simulink model "Plateforme_Stewart_fermeture_geometrique"  (R2019b)
settings: Solver=VariableStepAuto  StartTime=0.0  StopTime=10.0  RelTol=1e-3
PreLoadFcn:
  | addpath('Simscape')
model workspace (MATLAB code in the model file):
  | % Simscape(TM) Multibody(TM) version: 7.0
  | 
  | % This is a model data file derived from a Simscape Multibody Import XML file using the smimport function.
  | % The data in this file sets the block parameter values in an imported Simscape Multibody model.
  | % For more information on this file, see the smimport function help page in the Simscape Multibody documentation.
  | % You can modify numerical values, but avoid any other changes to this file.
  | % Do not add code to this file. Do not edit the physical units shown in comments.
  | 
  | %%%VariableName:smiData
  | 
  | 
  | %============= RigidTransform =============%
  | 
  | %Initialize the RigidTransform structure array by filling in null values.
  | smiData.RigidTransform(118).translation = [0.0 0.0 0.0];
  | smiData.RigidTransform(118).angle = 0.0;
  | smiData.RigidTransform(118).axis = [0.0 0.0 0.0];
  | smiData.RigidTransform(118).ID = '';
  | 
  | %Translation Method - Cartesian
  | %Rotation Method - Arbitrary Axis
  | smiData.RigidTransform(1).translation = [-109.40044094211088 0 0];  % mm
  | smiData.RigidTransform(1).angle = 0;  % rad
  | smiData.RigidTransform(1).axis = [0 0 0];
  | smiData.RigidTransform(1).ID = 'B[tige_verin-1:-:table_pltf-1]';
  | 
  | %Translation Method - Cartesian
  | %Rotation Method - Arbitrary Axis
  | smiData.RigidTransform(2).translation = [-577.50595932455826 -145.286666388404 9.0000000000001101];  % mm
  | smiData.RigidTransform(2).angle = 0;  % rad
  | smiData.RigidTransform(2).axis = [0 0 0];
  | smiData.RigidTransform(2).ID = 'F[tige_verin-1:-:table_pltf-1]';
  | 
  | %Translation Method - Cartesian
  | %Rotation Method - Arbitrary Axis
  | smiData.RigidTransform(3).translation = [-109.40044094211093 0 0];  % mm
  | smiData.RigidTransform(3).angle = 0;  % rad
  | smiData.RigidTransform(3).axis = [0 0 0];
  | smiData.RigidTransform(3).ID = 'B[tige_verin-2:-:table_pltf-1]';
  | 
  | %Translation Method - Cartesian
  | %Rotation Method - Arbitrary Axis
  | smiData.RigidTransform(4).translation = [-418.63100558659301 129.892825535908 9.0000000000000355];  % mm
  | smiData.RigidTransform(4).angle = 0;  % rad
  | smiData.RigidTransform(4).axis = [0 0 0];
  | smiData.RigidTransform(4).ID = 'F[tige_verin-2:-:table_pltf-1]';
  | 
  | %Translation Method - Cartesian
  | %Rotation Method - Arbitrary Axis
  | smiData.RigidTransform(5).translation = [-109.40044094211082 0 0];  % mm
  | smiData.RigidTransform(5).angle = 0;  % rad
  | smiData.RigidTransform(5).axis = [0 0 0];
  | smiData.RigidTransform(5).ID = 'B[tige_verin-4:-:table_pltf-1]';
  | 
  | %Translation Method - Cartesian
  | %Rotation Method - Arbitrary Axis
  | smiData.RigidTransform(6).translation = [-378.63100558659278 129.892825535908 9.0000000000002593];  % mm
  | smiData.RigidTransform(6).angle = 0;  % rad
  | smiData.RigidTransform(6).axis = [0 0 0];
  | smiData.RigidTransform(6).ID = 'F[tige_verin-4:-:table_pltf-1]';
  | 
  | %Translation Method - Cartesian
  | %Rotation Method - Arbitrary Axis
  | smiData.RigidTransform(7).translation = [-109.40044094211088 0 0];  % mm
  | smiData.RigidTransform(7).angle = 0;  % rad
  | smiData.RigidTransform(7).axis = [0 0 0];
  | smiData.RigidTransform(7).ID = 'B[tige_verin-5:-:table_pltf-1]';
  | 
  | %Translation Method - Cartesian
  | %Rotation Method - Arbitrary Axis
  | smiData.RigidTransform(8).translation = [-219.75605184862661 -145.28666638840158 9.0000000000000586];  % mm
  | smiData.RigidTransform(8).angle = 0;  % rad
  | smiData.RigidTransform(8).axis = [0 0 0];
  | smiData.RigidTransform(8).ID = 'F[tige_verin-5:-:table_pltf-1]';
  | 
  | %Translation Method - Cartesian
  | %Rotation Method - Arbitrary Axis
  | smiData.RigidTransform(9).translation = [-109.40044094211088 0 0];  % mm
  | smiData.RigidTransform(9).angle = 0;  % rad
  | smiData.RigidTransform(9).axis = [0 0 0];
  | smiData.RigidTransform(9).ID = 'B[tige_verin-6:-:table_pltf-1]';
  | 
  | %Translation Method - Cartesian
  | %Rotation Method - Arbitrary Axis
  | smiData.RigidTransform(10).translation = [-239.7560518486261 -179.92768253977937 9.0000000000000817];  % mm
  | smiData.RigidTransform(10).angle = 0;  % rad
  | smiData.RigidTransform(10).axis = [0 0 0];
  | smiData.RigidTransform(10).ID = 'F[tige_verin-6:-:table_pltf-1]';
  | 
  | %Translation Method - Cartesian
  | %Rotation Method - Arbitrary Axis
  | smiData.RigidTransform(11).translation = [-109.40044094211082 0 0];  % mm
  | smiData.RigidTransform(11).angle = 0;  % rad
  | smiData.RigidTransform(11).axis = [0 0 0];
  | smiData.RigidTransform(11).ID = 'B[tige_verin-7:-:table_pltf-1]';
  | 
  | %Translation Method - Cartesian
  | %Rotation Method - Arbitrary Axis
  | smiData.RigidTransform(12).translation = [-557.50595932455781 -179.92768253978147 9.0000000000000728];  % mm
  | smiData.RigidTransform(12).angle = 0;  % rad
  | smiData.RigidTransform(12).axis = [0 0 0];
  | smiData.RigidTransform(12).ID = 'F[tige_verin-7:-:table_pltf-1]';
  | 
  | %Translation Method - Cartesian
  | %Rotation Method - Arbitrary Axis
  | smiData.RigidTransform(13).translation = [0 0 0];  % mm
  | smiData.RigidTransform(13).angle = 0;  % rad
  | smiData.RigidTransform(13).axis = [0 0 0];
  | smiData.RigidTransform(13).ID = 'B[embase_pltf-1:-:]';
  | 
  | %Translation Method - Cartesian
  | %Rotation Method - Arbitrary Axis
  | smiData.RigidTransform(14).translation = [0 0 0];  % mm
  | smiData.RigidTransform(14).angle = 3.1415926535897931;  % rad
  | smiData.RigidTransform(14).axis = [2.4146537633967791e-16 -1 1.716137840753504e-16];
  | smiData.RigidTransform(14).ID = 'F[embase_pltf-1:-:]';
  | 
  | %Translation Method - Cartesian
  | %Rotation Method - Arbitrary Axis
  | smiData.RigidTransform(15).translation = [-21.777181335342689 270.78500270056696 -10.421088649404936];  % mm
  | smiData.RigidTransform(15).angle = 0;  % rad
  | smiData.RigidTransform(15).axis = [0 0 0];
  | smiData.RigidTransform(15).ID = 'B[embase_pltf-1:-:corps_verin-1]';
  | 
  | %Translation Method - Cartesian
  | %Rotation Method - Arbitrary Axis
  | smiData.RigidTransform(16).translation = [-402.58704714007331 -133.73646344618052 13.096795646989449];  % mm
  | smiData.RigidTransform(16).angle = 0;  % rad
  | smiData.RigidTransform(16).axis = [0 0 0];
  | smiData.RigidTransform(16).ID = 'F[embase_pltf-1:-:corps_verin-1]';
  | 
  | %Translation Method - Cartesian
  | %Rotation Method - Arbitrary Axis
  | smiData.RigidTransform(17).translation = [20.111591903521756 272.65573361842087 -6.7232809872821688];  % mm
  | smiData.RigidTransform(17).angle = 0;  % rad
  | smiData.RigidTransform(17).axis = [0 0 0];
  | smiData.RigidTransform(17).ID = 'B[embase_pltf-1:-:corps_verin-2]';
  | 
  | %Translation Method - Cartesian
  | %Rotation Method - Arbitrary Axis
  | smiData.RigidTransform(18).translation = [-402.58704714007342 -133.73646344618064 13.096795646989392];  % mm
  | smiData.RigidTransform(18).angle = 0;  % rad
  | smiData.RigidTransform(18).axis = [0 0 0];
  | smiData.RigidTransform(18).ID = 'F[embase_pltf-1:-:corps_verin-2]';
  | 
  | %Translation Method - Cartesian
  | %Rotation Method - Arbitrary Axis
  | smiData.RigidTransform(19).translation = [246.18258775279722 -118.91071731021286 -6.7232809872821191];  % mm
  | smiData.RigidTransform(19).angle = 0;  % rad
  | smiData.RigidTransform(19).axis = [0 0 0];
  | smiData.RigidTransform(19).ID = 'B[embase_pltf-1:-:corps_verin-3]';
  | 
  | %Translation Method - Cartesian
  | %Rotation Method - Arbitrary Axis
  | smiData.RigidTransform(20).translation = [-402.58704714007342 -133.73646344617663 13.096795646991893];  % mm
  | smiData.RigidTransform(20).angle = 0;  % rad
  | smiData.RigidTransform(20).axis = [0 0 0];
  | smiData.RigidTransform(20).ID = 'F[embase_pltf-1:-:corps_verin-3]';
  | 
  | %Translation Method - Cartesian
  | %Rotation Method - Arbitrary Axis
  | smiData.RigidTransform(21).translation = [226.07099584927582 -153.74501630820362 -6.7232809872821164];  % mm
  | smiData.RigidTransform(21).angle = 0;  % rad
  | smiData.RigidTransform(21).axis = [0 0 0];
  | smiData.RigidTransform(21).ID = 'B[embase_pltf-1:-:corps_verin-4]';
  | 
  | %Translation Method - Cartesian
  | %Rotation Method - Arbitrary Axis
  | smiData.RigidTransform(22).translation = [-402.58704714007337 -133.73646344617981 13.096795646989108];  % mm
  | smiData.RigidTransform(22).angle = 0;  % rad
  | smiData.RigidTransform(22).axis = [0 0 0];
  | smiData.RigidTransform(22).ID = 'F[embase_pltf-1:-:corps_verin-4]';
  | 
  | %Translation Method - Cartesian
  | %Rotation Method - Arbitrary Axis
  | smiData.RigidTransform(23).translation = [-226.07099584927371 -153.74501630820677 -6.7232809872821617];  % mm
  | smiData.RigidTransform(23).angle = 0;  % rad
  | smiData.RigidTransform(23).axis = [0 0 0];
  | smiData.RigidTransform(23).ID = 'B[embase_pltf-1:-:corps_verin-5]';
  | 
  | %Translation Method - Cartesian
  | %Rotation Method - Arbitrary Axis
  | smiData.RigidTransform(24).translation = [-402.58704714007354 -133.73646344618081 13.096795646989619];  % mm
  | smiData.RigidTransform(24).angle = 0;  % rad
  | smiData.RigidTransform(24).axis = [0 0 0];
  | smiData.RigidTransform(24).ID = 'F[embase_pltf-1:-:corps_verin-5]';
  | 
  | %Translation Method - Cartesian
  | %Rotation Method - Arbitrary Axis
  | smiData.RigidTransform(25).translation = [-246.18258775279565 -118.91071731021631 -6.7232809872821564];  % mm
  | smiData.RigidTransform(25).angle = 0;  % rad
  | smiData.RigidTransform(25).axis = [0 0 0];
  | smiData.RigidTransform(25).ID = 'B[embase_pltf-1:-:corps_verin-6]';
  | 
  | %Translation Method - Cartesian
  | %Rotation Method - Arbitrary Axis
  | smiData.RigidTransform(26).translation = [-402.58704714007354 -133.73646344618049 13.096795646989506];  % mm
  | smiData.RigidTransform(26).angle = 0;  % rad
  | smiData.RigidTransform(26).axis = [0 0 0];
  | smiData.RigidTransform(26).ID = 'F[embase_pltf-1:-:corps_verin-6]';
  | 
  | %Translation Method - Cartesian
  | %Rotation Method - Arbitrary Axis
  | smiData.RigidTransform(27).translation = [-258.58704714007337 -133.73646344618055 13.096795646989408];  % mm
  | smiData.RigidTransform(27).angle = 2.0943951023931953;  % rad
  | smiData.RigidTransform(27).axis = [-0.57735026918962584 -0.57735026918962584 0.57735026918962584];
  | smiData.RigidTransform(27).ID = 'B[corps_verin-1:-:tige_verin-1]';
  | 
  | %Translation Method - Cartesian
  | %Rotation Method - Arbitrary Axis
  | smiData.RigidTransform(28).translation = [-392.59341329234132 -3.1263880373444408e-13 1.1368683772161603e-13];  % mm
  | smiData.RigidTransform(28).angle = 2.0943951023931962;  % rad
  | smiData.RigidTransform(28).axis = [-0.57735026918962562 -0.57735026918962595 0.57735026918962573];
  | smiData.RigidTransform(28).ID = 'F[corps_verin-1:-:tige_verin-1]';
  | 
  | %Translation Method - Cartesian
  | %Rotation Method - Arbitrary Axis
  | smiData.RigidTransform(29).translation = [-258.58704714007342 -133.73646344618055 13.096795646989484];  % mm
  | smiData.RigidTransform(29).angle = 2.0943951023931953;  % rad
  | smiData.RigidTransform(29).axis = [-0.57735026918962584 -0.57735026918962584 0.57735026918962584];
  | smiData.RigidTransform(29).ID = 'B[corps_verin-2:-:tige_verin-2]';
  | 
  | %Translation Method - Cartesian
  | %Rotation Method - Arbitrary Axis
  | smiData.RigidTransform(30).translation = [-392.59341329234149 4.2632564145606011e-13 2.2737367544323206e-13];  % mm
  | smiData.RigidTransform(30).angle = 2.0943951023931944;  % rad
  | smiData.RigidTransform(30).axis = [-0.57735026918962595 -0.57735026918962529 0.57735026918962595];
  | smiData.RigidTransform(30).ID = 'F[corps_verin-2:-:tige_verin-2]';
  | 
  | %Translation Method - Cartesian
  | %Rotation Method - Arbitrary Axis
  | smiData.RigidTransform(31).translation = [-258.58704714007342 -133.73646344618058 13.096795646989456];  % mm
  | smiData.RigidTransform(31).angle = 2.0943951023931953;  % rad
  | smiData.RigidTransform(31).axis = [-0.57735026918962584 -0.57735026918962584 0.57735026918962584];
  | smiData.RigidTransform(31).ID = 'B[corps_verin-3:-:tige_verin-4]';
  | 
  | %Translation Method - Cartesian
  | %Rotation Method - Arbitrary Axis
  | smiData.RigidTransform(32).translation = [-392.59341329234132 -4.2916781239910051e-12 1.0231815394945443e-12];  % mm
  | smiData.RigidTransform(32).angle = 2.0943951023931953;  % rad
  | smiData.RigidTransform(32).axis = [-0.57735026918962629 -0.57735026918962584 0.57735026918962529];
  | smiData.RigidTransform(32).ID = 'F[corps_verin-3:-:tige_verin-4]';
  | 
  | %Translation Method - Cartesian
  | %Rotation Method - Arbitrary Axis
  | smiData.RigidTransform(33).translation = [-258.58704714007342 -133.73646344618061 13.096795646989429];  % mm
  | smiData.RigidTransform(33).angle = 2.0943951023931953;  % rad
  | smiData.RigidTransform(33).axis = [-0.57735026918962584 -0.57735026918962584 0.57735026918962584];
  | smiData.RigidTransform(33).ID = 'B[corps_verin-4:-:tige_verin-5]';
  | 
  | %Translation Method - Cartesian
  | %Rotation Method - Arbitrary Axis
  | smiData.RigidTransform(34).translation = [-392.59341329234155 8.6686213762732223e-13 6.8212102632969618e-13];  % mm
  | smiData.RigidTransform(34).angle = 2.0943951023931948;  % rad
  | smiData.RigidTransform(34).axis = [-0.57735026918962529 -0.57735026918962551 0.57735026918962662];
  | smiData.RigidTransform(34).ID = 'F[corps_verin-4:-:tige_verin-5]';
  | 
  | %Translation Method - Cartesian
  | %Rotation Method - Arbitrary Axis
  | smiData.RigidTransform(35).translation = [-258.58704714007331 -133.73646344618061 13.096795646989477];  % mm
  | smiData.RigidTransform(35).angle = 2.0943951023931953;  % rad
  | smiData.RigidTransform(35).axis = [-0.57735026918962584 -0.57735026918962584 0.57735026918962584];
  | smiData.RigidTransform(35).ID = 'B[corps_verin-5:-:tige_verin-6]';
  | 
  | %Translation Method - Cartesian
  | %Rotation Method - Arbitrary Axis
  | smiData.RigidTransform(36).translation = [-392.59341329234189 1.4210854715202004e-13 2.2737367544323206e-13];  % mm
  | smiData.RigidTransform(36).angle = 2.0943951023931953;  % rad
  | smiData.RigidTransform(36).axis = [-0.57735026918962618 -0.57735026918962562 0.5773502691896254];
  | smiData.RigidTransform(36).ID = 'F[corps_verin-5:-:tige_verin-6]';
  | 
  | %Translation Method - Cartesian
  | %Rotation Method - Arbitrary Axis
  | smiData.RigidTransform(37).translation = [-258.58704714007342 -133.73646344618055 13.096795646989401];  % mm
  | smiData.RigidTransform(37).angle = 2.0943951023931953;  % rad
  | smiData.RigidTransform(37).axis = [-0.57735026918962584 -0.57735026918962584 0.57735026918962584];
  | smiData.RigidTransform(37).ID = 'B[corps_verin-6:-:tige_verin-7]';
  | 
  | %Translation Method - Cartesian
  | %Rotation Method - Arbitrary Axis
  | smiData.RigidTransform(38).translation = [-392.59341329234144 1.9895196601282805e-13 -2.2737367544323206e-13];  % mm
  | smiData.RigidTransform(38).angle = 2.0943951023931953;  % rad
  | smiData.RigidTransform(38).axis = [-0.57735026918962595 -0.57735026918962562 0.57735026918962562];
  | smiData.RigidTransform(38).ID = 'F[corps_verin-6:-:tige_verin-7]';
  | 
  | %Translation Method - Cartesian
  | %Rotation Method - Arbitrary Axis
  | smiData.RigidTransform(39).translation = [-385.58704714007331 -133.73646344618061 13.096795646989415];  % mm
  | smiData.RigidTransform(39).angle = 0;  % rad
  | smiData.RigidTransform(39).axis = [0 0 0];
  | smiData.RigidTransform(39).ID = 'AssemblyGround[corps_verin-1:tube_inf-1]';
  | 
  | %Translation Method - Cartesian
  | %Rotation Method - Arbitrary Axis
  | smiData.RigidTransform(40).translation = [-385.58704714007342 -133.73646344618055 13.096795646989401];  % mm
  | smiData.RigidTransform(40).angle = 0;  % rad
  | smiData.RigidTransform(40).axis = [0 0 0];
  | smiData.RigidTransform(40).ID = 'AssemblyGround[corps_verin-1:embout_inf-1]';
  | 
  | %Translation Method - Cartesian
  | %Rotation Method - Arbitrary Axis
  | smiData.RigidTransform(41).translation = [-402.58704714007337 -133.73646344618055 13.096795646989394];  % mm
  | smiData.RigidTransform(41).angle = 0;  % rad
  | smiData.RigidTransform(41).axis = [0 0 0];
  | smiData.RigidTransform(41).ID = 'AssemblyGround[corps_verin-1:sphere-1]';
  | 
  | %Translation Method - Cartesian
  | %Rotation Method - Arbitrary Axis
  | smiData.RigidTransform(42).translation = [-271.58704714007337 -133.73646344618061 13.096795646989401];  % mm
  | smiData.RigidTransform(42).angle = 0;  % rad
  | smiData.RigidTransform(42).axis = [0 0 0];
  | smiData.RigidTransform(42).ID = 'AssemblyGround[corps_verin-1:boitier-1]';
  | 
  | %Translation Method - Cartesian
  | %Rotation Method - Arbitrary Axis
  | smiData.RigidTransform(43).translation = [-258.58704714007337 -133.73646344618055 13.096795646989408];  % mm
  | smiData.RigidTransform(43).angle = 0;  % rad
  | smiData.RigidTransform(43).axis = [0 0 0];
  | smiData.RigidTransform(43).ID = 'AssemblyGround[corps_verin-1:tube_sup-1]';
  | 
  | %Translation Method - Cartesian
  | %Rotation Method - Arbitrary Axis
  | smiData.RigidTransform(44).translation = [-271.58704714007337 -117.73646344618061 6.8467956469894027];  % mm
  | smiData.RigidTransform(44).angle = 1.5707963267948966;  % rad
  | smiData.RigidTransform(44).axis = [-1 -1.3877787807814457e-16 -1.3877787807814467e-16];
  | smiData.RigidTransform(44).ID = 'AssemblyGround[corps_verin-1:couvercle-1]';
  | 
  | %Translation Method - Cartesian
  | %Rotation Method - Arbitrary Axis
  | smiData.RigidTransform(45).translation = [-47.394074789842975 -133.73646344618061 13.096795646989456];  % mm
  | smiData.RigidTransform(45).angle = 3.1415926535897931;  % rad
  | smiData.RigidTransform(45).axis = [-2.851611096621234e-17 0.22941107115039033 0.97332962578647042];
  | smiData.RigidTransform(45).ID = 'AssemblyGround[corps_verin-1:palier-1]';
  | 
  | %Translation Method - Cartesian
  | %Rotation Method - Arbitrary Axis
  | smiData.RigidTransform(46).translation = [-121.40044094211083 0 0];  % mm
  | smiData.RigidTransform(46).angle = 3.1415926535897931;  % rad
  | smiData.RigidTransform(46).axis = [6.3638526192303913e-17 0.47606521271394214 0.87940998018195637];
  | smiData.RigidTransform(46).ID = 'AssemblyGround[tige_verin-7:embout_sup-1]';
  | 
  | %Translation Method - Cartesian
  | %Rotation Method - Arbitrary Axis
  | smiData.RigidTransform(47).translation = [-281.40044094211089 0 0];  % mm
  | smiData.RigidTransform(47).angle = 0.80510609664977162;  % rad
  | smiData.RigidTransform(47).axis = [-1 0 0];
  | smiData.RigidTransform(47).ID = 'AssemblyGround[tige_verin-7:tige-1]';
  | 
  | %Translation Method - Cartesian
  | %Rotation Method - Arbitrary Axis
  | smiData.RigidTransform(48).translation = [-286.40044094211095 0 0];  % mm
  | smiData.RigidTransform(48).angle = 0;  % rad
  | smiData.RigidTransform(48).axis = [0 0 0];
  | smiData.RigidTransform(48).ID = 'AssemblyGround[tige_verin-7:ecrou-1]';
  | 
  | %Translation Method - Cartesian
  | %Rotation Method - Arbitrary Axis
  | smiData.RigidTransform(49).translation = [-109.40044094211082 0 0];  % mm
  | smiData.RigidTransform(49).angle = 0;  % rad
  | smiData.RigidTransform(49).axis = [0 0 0];
  | smiData.RigidTransform(49).ID = 'AssemblyGround[tige_verin-7:sphere-1]';
  | 
  | %Translation Method - Cartesian
  | %Rotation Method - Arbitrary Axis
  | smiData.RigidTransform(50).translation = [-238.63105184862621 -177.9791253812642 5.1028856829702374];  % mm
  | smiData.RigidTransform(50).angle = 1.8452184908695632;  % rad
  | smiData.RigidTransform(50).axis = [0.12851178747769235 -0.94870612275177946 -0.28886227364017958];
  | smiData.RigidTransform(50).ID = 'AssemblyGround[table_pltf-1:ext_sph-6]';
  | 
  | %Translation Method - Cartesian
  | %Rotation Method - Arbitrary Axis
  | smiData.RigidTransform(51).translation = [-558.63095932455781 -177.97912538126641 5.1028856829702374];  % mm
  | smiData.RigidTransform(51).angle = 1.3181160716528153;  % rad
  | smiData.RigidTransform(51).axis = [8.5997505698985228e-17 -0.89442719099991586 -0.44721359549995787];
  | smiData.RigidTransform(51).ID = 'AssemblyGround[table_pltf-1:ext_sph-4]';
  | 
  | %Translation Method - Cartesian
  | %Rotation Method - Arbitrary Axis
  | smiData.RigidTransform(52).translation = [-416.38100558659278 129.89282553590814 5.1028856829702374];  % mm
  | smiData.RigidTransform(52).angle = 1.1138509682631477;  % rad
  | smiData.RigidTransform(52).axis = [-0.32436275744359122 0.92721000971271517 0.18727092532514639];
  | smiData.RigidTransform(52).ID = 'AssemblyGround[table_pltf-1:ext_sph-1]';
  | 
  | %Translation Method - Cartesian
  | %Rotation Method - Arbitrary Axis
  | smiData.RigidTransform(53).translation = [-220.88105184862647 -147.23522354691647 5.1028856829702924];  % mm
  | smiData.RigidTransform(53).angle = 1.4414924728059237;  % rad
  | smiData.RigidTransform(53).axis = [-0.37279524950071685 -0.91787977789370334 0.13608973246907444];
  | smiData.RigidTransform(53).ID = 'AssemblyGround[table_pltf-1:ext_sph-5]';
  | 
  | %Translation Method - Cartesian
  | %Rotation Method - Arbitrary Axis
  | smiData.RigidTransform(54).translation = [-380.88100558659272 129.89282553590814 5.1028856829703484];  % mm
  | smiData.RigidTransform(54).angle = 1.3047235338847067;  % rad
  | smiData.RigidTransform(54).axis = [-0.56711997758819543 -0.75575563159914327 -0.32742687172335888];
  | smiData.RigidTransform(54).ID = 'AssemblyGround[table_pltf-1:ext_sph-2]';
  | 
  | %Translation Method - Cartesian
  | %Rotation Method - Arbitrary Axis
  | smiData.RigidTransform(55).translation = [-576.38095932455803 -147.23522354691895 5.1028856829701823];  % mm
  | smiData.RigidTransform(55).angle = 1.5789537349491201;  % rad
  | smiData.RigidTransform(55).axis = [-0.5060320994735239 0.86248629273953803 0.006993506904675686];
  | smiData.RigidTransform(55).ID = 'AssemblyGround[table_pltf-1:ext_sph-3]';
  | 
  | %Translation Method - Cartesian
  | %Rotation Method - Arbitrary Axis
  | smiData.RigidTransform(56).translation = [-398.63100558659278 -65.107174464091898 -12.547005383792332];  % mm
  | smiData.RigidTransform(56).angle = 0;  % rad
  | smiData.RigidTransform(56).axis = [0 0 0];
  | smiData.RigidTransform(56).ID = 'AssemblyGround[table_pltf-1:table3-1]';
  | 
  | %Translation Method - Cartesian
  | %Rotation Method - Arbitrary Axis
  | smiData.RigidTransform(57).translation = [-385.58704714007331 -133.73646344618061 13.096795646989456];  % mm
  | smiData.RigidTransform(57).angle = 0;  % rad
  | smiData.RigidTransform(57).axis = [0 0 0];
  | smiData.RigidTransform(57).ID = 'AssemblyGround[corps_verin-3:tube_inf-1]';
  | 
  | %Translation Method - Cartesian
  | %Rotation Method - Arbitrary Axis
  | smiData.RigidTransform(58).translation = [-385.58704714007342 -133.73646344618061 13.096795646989456];  % mm
  | smiData.RigidTransform(58).angle = 0;  % rad
  | smiData.RigidTransform(58).axis = [0 0 0];
  | smiData.RigidTransform(58).ID = 'AssemblyGround[corps_verin-3:embout_inf-1]';
  | 
  | %Translation Method - Cartesian
  | %Rotation Method - Arbitrary Axis
  | smiData.RigidTransform(59).translation = [-402.58704714007337 -133.73646344618061 13.096795646989456];  % mm
  | smiData.RigidTransform(59).angle = 0;  % rad
  | smiData.RigidTransform(59).axis = [0 0 0];
  | smiData.RigidTransform(59).ID = 'AssemblyGround[corps_verin-3:sphere-1]';
  | 
  | %Translation Method - Cartesian
  | %Rotation Method - Arbitrary Axis
  | smiData.RigidTransform(60).translation = [-271.58704714007337 -133.73646344618058 13.096795646989484];  % mm
  | smiData.RigidTransform(60).angle = 0;  % rad
  | smiData.RigidTransform(60).axis = [0 0 0];
  | smiData.RigidTransform(60).ID = 'AssemblyGround[corps_verin-3:boitier-1]';
  | 
  | %Translation Method - Cartesian
  | %Rotation Method - Arbitrary Axis
  | smiData.RigidTransform(61).translation = [-258.58704714007342 -133.73646344618058 13.096795646989456];  % mm
  | smiData.RigidTransform(61).angle = 0;  % rad
  | smiData.RigidTransform(61).axis = [0 0 0];
  | smiData.RigidTransform(61).ID = 'AssemblyGround[corps_verin-3:tube_sup-1]';
  | 
  | %Translation Method - Cartesian
  | %Rotation Method - Arbitrary Axis
  | smiData.RigidTransform(62).translation = [-271.58704714007331 -117.73646344618059 6.8467956469894506];  % mm
  | smiData.RigidTransform(62).angle = 1.5707963267948966;  % rad
  | smiData.RigidTransform(62).axis = [-1 -9.7144514654701185e-17 -1.2490009027033011e-16];
  | smiData.RigidTransform(62).ID = 'AssemblyGround[corps_verin-3:couvercle-1]';
  | 
  | %Translation Method - Cartesian
  | %Rotation Method - Arbitrary Axis
  | smiData.RigidTransform(63).translation = [-47.394074789842975 -133.73646344618066 13.096795646989484];  % mm
  | smiData.RigidTransform(63).angle = 3.1415926535897931;  % rad
  | smiData.RigidTransform(63).axis = [3.1848379601679358e-17 0.22941107115039044 0.97332962578647042];
  | smiData.RigidTransform(63).ID = 'AssemblyGround[corps_verin-3:palier-1]';
  | 
  | %Translation Method - Cartesian
  | %Rotation Method - Arbitrary Axis
  | smiData.RigidTransform(64).translation = [-385.58704714007337 -133.73646344618064 13.096795646989429];  % mm
  | smiData.RigidTransform(64).angle = 0;  % rad
  | smiData.RigidTransform(64).axis = [0 0 0];
  | smiData.RigidTransform(64).ID = 'AssemblyGround[corps_verin-4:tube_inf-1]';
  | 
  | %Translation Method - Cartesian
  | %Rotation Method - Arbitrary Axis
  | smiData.RigidTransform(65).translation = [-385.58704714007348 -133.73646344618066 13.096795646989456];  % mm
  | smiData.RigidTransform(65).angle = 0;  % rad
  | smiData.RigidTransform(65).axis = [0 0 0];
  | smiData.RigidTransform(65).ID = 'AssemblyGround[corps_verin-4:embout_inf-1]';
  | 
  | %Translation Method - Cartesian
  | %Rotation Method - Arbitrary Axis
  | smiData.RigidTransform(66).translation = [-402.58704714007342 -133.73646344618061 13.096795646989456];  % mm
  | smiData.RigidTransform(66).angle = 0;  % rad
  | smiData.RigidTransform(66).axis = [0 0 0];
  | smiData.RigidTransform(66).ID = 'AssemblyGround[corps_verin-4:sphere-1]';
  | 
  | %Translation Method - Cartesian
  | %Rotation Method - Arbitrary Axis
  | smiData.RigidTransform(67).translation = [-271.58704714007337 -133.73646344618066 13.096795646989429];  % mm
  | smiData.RigidTransform(67).angle = 0;  % rad
  | smiData.RigidTransform(67).axis = [0 0 0];
  | smiData.RigidTransform(67).ID = 'AssemblyGround[corps_verin-4:boitier-1]';
  | 
  | %Translation Method - Cartesian
  | %Rotation Method - Arbitrary Axis
  | smiData.RigidTransform(68).translation = [-258.58704714007342 -133.73646344618061 13.096795646989429];  % mm
  | smiData.RigidTransform(68).angle = 0;  % rad
  | smiData.RigidTransform(68).axis = [0 0 0];
  | smiData.RigidTransform(68).ID = 'AssemblyGround[corps_verin-4:tube_sup-1]';
  | 
  | %Translation Method - Cartesian
  | %Rotation Method - Arbitrary Axis
  | smiData.RigidTransform(69).translation = [-271.58704714007337 -117.73646344618064 6.8467956469894231];  % mm
  | smiData.RigidTransform(69).angle = 1.5707963267948966;  % rad
  | smiData.RigidTransform(69).axis = [-1 -1.1796119636642288e-16 -2.4980018054066022e-16];
  | smiData.RigidTransform(69).ID = 'AssemblyGround[corps_verin-4:couvercle-1]';
  | 
  | %Translation Method - Cartesian
  | %Rotation Method - Arbitrary Axis
  | smiData.RigidTransform(70).translation = [-47.394074789843032 -133.73646344618066 13.096795646989429];  % mm
  | smiData.RigidTransform(70).angle = 3.1415926535897931;  % rad
  | smiData.RigidTransform(70).axis = [2.8516110966212334e-17 0.22941107115039044 0.97332962578647042];
  | smiData.RigidTransform(70).ID = 'AssemblyGround[corps_verin-4:palier-1]';
  | 
  | %Translation Method - Cartesian
  | %Rotation Method - Arbitrary Axis
  | smiData.RigidTransform(71).translation = [-121.40044094211089 0 0];  % mm
  | smiData.RigidTransform(71).angle = 3.1415926535897931;  % rad
  | smiData.RigidTransform(71).axis = [0 0.4760652127139422 0.8794099801819566];
  | smiData.RigidTransform(71).ID = 'AssemblyGround[tige_verin-5:embout_sup-1]';
  | 
  | %Translation Method - Cartesian
  | %Rotation Method - Arbitrary Axis
  | smiData.RigidTransform(72).translation = [-281.40044094211089 0 0];  % mm
  | smiData.RigidTransform(72).angle = 0.80510609664977162;  % rad
  | smiData.RigidTransform(72).axis = [-1 -2.5106205397484075e-16 7.700212191956017e-17];
  | smiData.RigidTransform(72).ID = 'AssemblyGround[tige_verin-5:tige-1]';
  | 
  | %Translation Method - Cartesian
  | %Rotation Method - Arbitrary Axis
  | smiData.RigidTransform(73).translation = [-286.40044094211095 0 0];  % mm
  | smiData.RigidTransform(73).angle = 0;  % rad
  | smiData.RigidTransform(73).axis = [0 0 0];
  | smiData.RigidTransform(73).ID = 'AssemblyGround[tige_verin-5:ecrou-1]';
  | 
  | %Translation Method - Cartesian
  | %Rotation Method - Arbitrary Axis
  | smiData.RigidTransform(74).translation = [-109.40044094211088 0 0];  % mm
  | smiData.RigidTransform(74).angle = 0;  % rad
  | smiData.RigidTransform(74).axis = [0 0 0];
  | smiData.RigidTransform(74).ID = 'AssemblyGround[tige_verin-5:sphere-1]';
  | 
  | %Translation Method - Cartesian
  | %Rotation Method - Arbitrary Axis
  | smiData.RigidTransform(75).translation = [0 0 0];  % mm
  | smiData.RigidTransform(75).angle = 0;  % rad
  | smiData.RigidTransform(75).axis = [0 0 0];
  | smiData.RigidTransform(75).ID = 'AssemblyGround[embase_pltf-1:embase-1]';
  | 
  | %Translation Method - Cartesian
  | %Rotation Method - Arbitrary Axis
  | smiData.RigidTransform(76).translation = [-20.111591903521784 272.65573361842087 -6.7232809872821715];  % mm
  | smiData.RigidTransform(76).angle = 1.1886358755650654;  % rad
  | smiData.RigidTransform(76).axis = [-2.3930801898784881e-16 -0.89231044576403895 0.45142227280051467];
  | smiData.RigidTransform(76).ID = 'AssemblyGround[embase_pltf-1:ext_sph-1]';
  | 
  | %Translation Method - Cartesian
  | %Rotation Method - Arbitrary Axis
  | smiData.RigidTransform(77).translation = [20.111591903521756 272.65573361842087 -6.7232809872821688];  % mm
  | smiData.RigidTransform(77).angle = 1.1886358755650657;  % rad
  | smiData.RigidTransform(77).axis = [2.9913502373481095e-17 0.89231044576403895 -0.45142227280051433];
  | smiData.RigidTransform(77).ID = 'AssemblyGround[embase_pltf-1:ext_sph-2]';
  | 
  | %Translation Method - Cartesian
  | %Rotation Method - Arbitrary Axis
  | smiData.RigidTransform(78).translation = [246.18258775279722 -118.91071731021286 -6.7232809872821191];  % mm
  | smiData.RigidTransform(78).angle = 1.3935923944935191;  % rad
  | smiData.RigidTransform(78).axis = [5.6394261391252521e-17 -0.84111161395084555 -0.54086158384285687];
  | smiData.RigidTransform(78).ID = 'AssemblyGround[embase_pltf-1:ext_sph-3]';
  | 
  | %Translation Method - Cartesian
  | %Rotation Method - Arbitrary Axis
  | smiData.RigidTransform(79).translation = [226.07099584927582 -153.74501630820362 -6.7232809872821164];  % mm
  | smiData.RigidTransform(79).angle = 0.98938499076868036;  % rad
  | smiData.RigidTransform(79).axis = [-2.9061226051580059e-17 -0.99072835303675166 0.13585775829552582];
  | smiData.RigidTransform(79).ID = 'AssemblyGround[embase_pltf-1:ext_sph-4]';
  | 
  | %Translation Method - Cartesian
  | %Rotation Method - Arbitrary Axis
  | smiData.RigidTransform(80).translation = [-246.18258775279565 -118.91071731021631 -6.7232809872821564];  % mm
  | smiData.RigidTransform(80).angle = 1.3937057673028201;  % rad
  | smiData.RigidTransform(80).axis = [-0.011638836419521733 0.83574692275854157 0.54899145584100639];
  | smiData.RigidTransform(80).ID = 'AssemblyGround[embase_pltf-1:ext_sph-6]';
  | 
  | %Translation Method - Cartesian
  | %Rotation Method - Arbitrary Axis
  | smiData.RigidTransform(81).translation = [-226.07099584927371 -153.74501630820677 -6.7232809872821617];  % mm
  | smiData.RigidTransform(81).angle = 0.98938499076867825;  % rad
  | smiData.RigidTransform(81).axis = [2.9061226051580096e-17 0.99072835303675288 -0.13585775829551691];
  | smiData.RigidTransform(81).ID = 'AssemblyGround[embase_pltf-1:ext_sph-5]';
  | 
  | %Translation Method - Cartesian
  | %Rotation Method - Arbitrary Axis
  | smiData.RigidTransform(82).translation = [-385.58704714007331 -133.73646344618061 13.096795646989408];  % mm
  | smiData.RigidTransform(82).angle = 0;  % rad
  | smiData.RigidTransform(82).axis = [0 0 0];
  | smiData.RigidTransform(82).ID = 'AssemblyGround[corps_verin-5:tube_inf-1]';
  | 
  | %Translation Method - Cartesian
  | %Rotation Method - Arbitrary Axis
  | smiData.RigidTransform(83).translation = [-385.58704714007331 -133.73646344618061 13.096795646989477];  % mm
  | smiData.RigidTransform(83).angle = 0;  % rad
  | smiData.RigidTransform(83).axis = [0 0 0];
  | smiData.RigidTransform(83).ID = 'AssemblyGround[corps_verin-5:embout_inf-1]';
  | 
  | %Translation Method - Cartesian
  | %Rotation Method - Arbitrary Axis
  | smiData.RigidTransform(84).translation = [-402.58704714007331 -133.73646344618061 13.096795646989429];  % mm
  | smiData.RigidTransform(84).angle = 0;  % rad
  | smiData.RigidTransform(84).axis = [0 0 0];
  | smiData.RigidTransform(84).ID = 'AssemblyGround[corps_verin-5:sphere-1]';
  | 
  | %Translation Method - Cartesian
  | %Rotation Method - Arbitrary Axis
  | smiData.RigidTransform(85).translation = [-271.58704714007325 -133.73646344618061 13.096795646989463];  % mm
  | smiData.RigidTransform(85).angle = 0;  % rad
  | smiData.RigidTransform(85).axis = [0 0 0];
  | smiData.RigidTransform(85).ID = 'AssemblyGround[corps_verin-5:boitier-1]';
  | 
  | %Translation Method - Cartesian
  | %Rotation Method - Arbitrary Axis
  | smiData.RigidTransform(86).translation = [-258.58704714007331 -133.73646344618061 13.096795646989477];  % mm
  | smiData.RigidTransform(86).angle = 0;  % rad
  | smiData.RigidTransform(86).axis = [0 0 0];
  | smiData.RigidTransform(86).ID = 'AssemblyGround[corps_verin-5:tube_sup-1]';
  | 
  | %Translation Method - Cartesian
  | %Rotation Method - Arbitrary Axis
  | smiData.RigidTransform(87).translation = [-271.58704714007331 -117.73646344618061 6.8467956469894649];  % mm
  | smiData.RigidTransform(87).angle = 1.5707963267948966;  % rad
  | smiData.RigidTransform(87).axis = [-1 -1.3877787807814459e-16 -1.3877787807814462e-16];
  | smiData.RigidTransform(87).ID = 'AssemblyGround[corps_verin-5:couvercle-1]';
  | 
  | %Translation Method - Cartesian
  | %Rotation Method - Arbitrary Axis
  | smiData.RigidTransform(88).translation = [-47.394074789843032 -133.73646344618066 13.096795646989499];  % mm
  | smiData.RigidTransform(88).angle = 3.1415926535897931;  % rad
  | smiData.RigidTransform(88).axis = [3.820461799426253e-17 0.22941107115039039 0.97332962578647042];
  | smiData.RigidTransform(88).ID = 'AssemblyGround[corps_verin-5:palier-1]';
  | 
  | %Translation Method - Cartesian
  | %Rotation Method - Arbitrary Axis
  | smiData.RigidTransform(89).translation = [-385.58704714007342 -133.73646344618055 13.096795646989429];  % mm
  | smiData.RigidTransform(89).angle = 0;  % rad
  | smiData.RigidTransform(89).axis = [0 0 0];
  | smiData.RigidTransform(89).ID = 'AssemblyGround[corps_verin-2:tube_inf-1]';
  | 
  | %Translation Method - Cartesian
  | %Rotation Method - Arbitrary Axis
  | smiData.RigidTransform(90).translation = [-385.58704714007354 -133.73646344618058 13.096795646989456];  % mm
  | smiData.RigidTransform(90).angle = 0;  % rad
  | smiData.RigidTransform(90).axis = [0 0 0];
  | smiData.RigidTransform(90).ID = 'AssemblyGround[corps_verin-2:embout_inf-1]';
  | 
  | %Translation Method - Cartesian
  | %Rotation Method - Arbitrary Axis
  | smiData.RigidTransform(91).translation = [-402.58704714007348 -133.73646344618055 13.096795646989513];  % mm
  | smiData.RigidTransform(91).angle = 0;  % rad
  | smiData.RigidTransform(91).axis = [0 0 0];
  | smiData.RigidTransform(91).ID = 'AssemblyGround[corps_verin-2:sphere-1]';
  | 
  | %Translation Method - Cartesian
  | %Rotation Method - Arbitrary Axis
  | smiData.RigidTransform(92).translation = [-271.58704714007342 -133.73646344618055 13.096795646989456];  % mm
  | smiData.RigidTransform(92).angle = 0;  % rad
  | smiData.RigidTransform(92).axis = [0 0 0];
  | smiData.RigidTransform(92).ID = 'AssemblyGround[corps_verin-2:boitier-1]';
  | 
  | %Translation Method - Cartesian
  | %Rotation Method - Arbitrary Axis
  | smiData.RigidTransform(93).translation = [-258.58704714007342 -133.73646344618055 13.096795646989484];  % mm
  | smiData.RigidTransform(93).angle = 0;  % rad
  | smiData.RigidTransform(93).axis = [0 0 0];
  | smiData.RigidTransform(93).ID = 'AssemblyGround[corps_verin-2:tube_sup-1]';
  | 
  | %Translation Method - Cartesian
  | %Rotation Method - Arbitrary Axis
  | smiData.RigidTransform(94).translation = [-271.58704714007337 -117.73646344618058 6.8467956469894506];  % mm
  | smiData.RigidTransform(94).angle = 1.5707963267948966;  % rad
  | smiData.RigidTransform(94).axis = [-1 -1.457167719820518e-16 -1.5265566588595902e-16];
  | smiData.RigidTransform(94).ID = 'AssemblyGround[corps_verin-2:couvercle-1]';
  | 
  | %Translation Method - Cartesian
  | %Rotation Method - Arbitrary Axis
  | smiData.RigidTransform(95).translation = [-47.394074789843032 -133.73646344618064 13.096795646989456];  % mm
  | smiData.RigidTransform(95).angle = 3.1415926535897931;  % rad
  | smiData.RigidTransform(95).axis = [0 0.22941107115039042 0.97332962578647042];
  | smiData.RigidTransform(95).ID = 'AssemblyGround[corps_verin-2:palier-1]';
  | 
  | %Translation Method - Cartesian
  | %Rotation Method - Arbitrary Axis
  | smiData.RigidTransform(96).translation = [-121.40044094211089 0 0];  % mm
  | smiData.RigidTransform(96).angle = 3.1415926535897931;  % rad
  | smiData.RigidTransform(96).axis = [0 0.4760652127139422 0.8794099801819566];
  | smiData.RigidTransform(96).ID = 'AssemblyGround[tige_verin-1:embout_sup-1]';
  | 
  | %Translation Method - Cartesian
  | %Rotation Method - Arbitrary Axis
  | smiData.RigidTransform(97).translation = [-281.40044094211089 0 0];  % mm
  | smiData.RigidTransform(97).angle = 0.80510609664977162;  % rad
  | smiData.RigidTransform(97).axis = [-1 0 0];
  | smiData.RigidTransform(97).ID = 'AssemblyGround[tige_verin-1:tige-1]';
  | 
  | %Translation Method - Cartesian
  | %Rotation Method - Arbitrary Axis
  | smiData.RigidTransform(98).translation = [-286.40044094211095 0 0];  % mm
  | smiData.RigidTransform(98).angle = 0;  % rad
  | smiData.RigidTransform(98).axis = [0 0 0];
  | smiData.RigidTransform(98).ID = 'AssemblyGround[tige_verin-1:ecrou-1]';
  | 
  | %Translation Method - Cartesian
  | %Rotation Method - Arbitrary Axis
  | smiData.RigidTransform(99).translation = [-109.40044094211088 0 0];  % mm
  | smiData.RigidTransform(99).angle = 0;  % rad
  | smiData.RigidTransform(99).axis = [0 0 0];
  | smiData.RigidTransform(99).ID = 'AssemblyGround[tige_verin-1:sphere-1]';
  | 
  | %Translation Method - Cartesian
  | %Rotation Method - Arbitrary Axis
  | smiData.RigidTransform(100).translation = [-121.40044094211083 0 0];  % mm
  | smiData.RigidTransform(100).angle = 3.1415926535897931;  % rad
  | smiData.RigidTransform(100).axis = [4.6111194121053712e-17 0.4760652127139422 0.87940998018195649];
  | smiData.RigidTransform(100).ID = 'AssemblyGround[tige_verin-6:embout_sup-1]';
  | 
  | %Translation Method - Cartesian
  | %Rotation Method - Arbitrary Axis
  | smiData.RigidTransform(101).translation = [-281.40044094211095 0 0];  % mm
  | smiData.RigidTransform(101).angle = 0.80510609664977162;  % rad
  | smiData.RigidTransform(101).axis = [-1 0 0];
  | smiData.RigidTransform(101).ID = 'AssemblyGround[tige_verin-6:tige-1]';
  | 
  | %Translation Method - Cartesian
  | %Rotation Method - Arbitrary Axis
  | smiData.RigidTransform(102).translation = [-286.40044094211095 0 0];  % mm
  | smiData.RigidTransform(102).angle = 0;  % rad
  | smiData.RigidTransform(102).axis = [0 0 0];
  | smiData.RigidTransform(102).ID = 'AssemblyGround[tige_verin-6:ecrou-1]';
  | 
  | %Translation Method - Cartesian
  | %Rotation Method - Arbitrary Axis
  | smiData.RigidTransform(103).translation = [-109.40044094211088 0 0];  % mm
  | smiData.RigidTransform(103).angle = 0;  % rad
  | smiData.RigidTransform(103).axis = [0 0 0];
  | smiData.RigidTransform(103).ID = 'AssemblyGround[tige_verin-6:sphere-1]';
  | 
  | %Translation Method - Cartesian
  | %Rotation Method - Arbitrary Axis
  | smiData.RigidTransform(104).translation = [-385.58704714007342 -133.73646344618052 13.096795646989429];  % mm
  | smiData.RigidTransform(104).angle = 0;  % rad
  | smiData.RigidTransform(104).axis = [0 0 0];
  | smiData.RigidTransform(104).ID = 'AssemblyGround[corps_verin-6:tube_inf-1]';
  | 
  | %Translation Method - Cartesian
  | %Rotation Method - Arbitrary Axis
  | smiData.RigidTransform(105).translation = [-385.58704714007348 -133.73646344618055 13.096795646989456];  % mm
  | smiData.RigidTransform(105).angle = 0;  % rad
  | smiData.RigidTransform(105).axis = [0 0 0];
  | smiData.RigidTransform(105).ID = 'AssemblyGround[corps_verin-6:embout_inf-1]';
  | 
  | %Translation Method - Cartesian
  | %Rotation Method - Arbitrary Axis
  | smiData.RigidTransform(106).translation = [-402.58704714007348 -133.73646344618052 13.096795646989401];  % mm
  | smiData.RigidTransform(106).angle = 0;  % rad
  | smiData.RigidTransform(106).axis = [0 0 0];
  | smiData.RigidTransform(106).ID = 'AssemblyGround[corps_verin-6:sphere-1]';
  | 
  | %Translation Method - Cartesian
  | %Rotation Method - Arbitrary Axis
  | smiData.RigidTransform(107).translation = [-271.58704714007342 -133.73646344618055 13.096795646989429];  % mm
  | smiData.RigidTransform(107).angle = 0;  % rad
  | smiData.RigidTransform(107).axis = [0 0 0];
  | smiData.RigidTransform(107).ID = 'AssemblyGround[corps_verin-6:boitier-1]';
  | 
  | %Translation Method - Cartesian
  | %Rotation Method - Arbitrary Axis
  | smiData.RigidTransform(108).translation = [-258.58704714007342 -133.73646344618055 13.096795646989401];  % mm
  | smiData.RigidTransform(108).angle = 0;  % rad
  | smiData.RigidTransform(108).axis = [0 0 0];
  | smiData.RigidTransform(108).ID = 'AssemblyGround[corps_verin-6:tube_sup-1]';
  | 
  | %Translation Method - Cartesian
  | %Rotation Method - Arbitrary Axis
  | smiData.RigidTransform(109).translation = [-271.58704714007342 -117.73646344618054 6.8467956469894231];  % mm
  | smiData.RigidTransform(109).angle = 1.5707963267948963;  % rad
  | smiData.RigidTransform(109).axis = [-1 -1.1102230246251568e-16 -2.5673907444456755e-16];
  | smiData.RigidTransform(109).ID = 'AssemblyGround[corps_verin-6:couvercle-1]';
  | 
  | %Translation Method - Cartesian
  | %Rotation Method - Arbitrary Axis
  | smiData.RigidTransform(110).translation = [-47.394074789843032 -133.73646344618064 13.096795646989401];  % mm
  | smiData.RigidTransform(110).angle = 3.1415926535897927;  % rad
  | smiData.RigidTransform(110).axis = [4.7761371462725099e-17 0.22941107115039042 0.97332962578647042];
  | smiData.RigidTransform(110).ID = 'AssemblyGround[corps_verin-6:palier-1]';
  | 
  | %Translation Method - Cartesian
  | %Rotation Method - Arbitrary Axis
  | smiData.RigidTransform(111).translation = [-121.40044094211095 0 0];  % mm
  | smiData.RigidTransform(111).angle = 3.1415926535897931;  % rad
  | smiData.RigidTransform(111).axis = [0 0.4760652127139422 0.87940998018195649];
  | smiData.RigidTransform(111).ID = 'AssemblyGround[tige_verin-2:embout_sup-1]';
  | 
  | %Translation Method - Cartesian
  | %Rotation Method - Arbitrary Axis
  | smiData.RigidTransform(112).translation = [-281.400440942111 0 0];  % mm
  | smiData.RigidTransform(112).angle = 0.80510609664977162;  % rad
  | smiData.RigidTransform(112).axis = [-1 0 0];
  | smiData.RigidTransform(112).ID = 'AssemblyGround[tige_verin-2:tige-1]';
  | 
  | %Translation Method - Cartesian
  | %Rotation Method - Arbitrary Axis
  | smiData.RigidTransform(113).translation = [-286.40044094211112 0 0];  % mm
  | smiData.RigidTransform(113).angle = 0;  % rad
  | smiData.RigidTransform(113).axis = [0 0 0];
  | smiData.RigidTransform(113).ID = 'AssemblyGround[tige_verin-2:ecrou-1]';
  | 
  | %Translation Method - Cartesian
  | %Rotation Method - Arbitrary Axis
  | smiData.RigidTransform(114).translation = [-109.40044094211093 0 0];  % mm
  | smiData.RigidTransform(114).angle = 0;  % rad
  | smiData.RigidTransform(114).axis = [0 0 0];
  | smiData.RigidTransform(114).ID = 'AssemblyGround[tige_verin-2:sphere-1]';
  | 
  | %Translation Method - Cartesian
  | %Rotation Method - Arbitrary Axis
  | smiData.RigidTransform(115).translation = [-121.40044094211083 0 0];  % mm
  | smiData.RigidTransform(115).angle = 3.1415926535897931;  % rad
  | smiData.RigidTransform(115).axis = [3.9451985196208029e-17 0.47606521271394209 0.87940998018195649];
  | smiData.RigidTransform(115).ID = 'AssemblyGround[tige_verin-4:embout_sup-1]';
  | 
  | %Translation Method - Cartesian
  | %Rotation Method - Arbitrary Axis
  | smiData.RigidTransform(116).translation = [-281.40044094211089 0 0];  % mm
  | smiData.RigidTransform(116).angle = 0.80510609664977162;  % rad
  | smiData.RigidTransform(116).axis = [-1 0 0];
  | smiData.RigidTransform(116).ID = 'AssemblyGround[tige_verin-4:tige-1]';
  | 
  | %Translation Method - Cartesian
  | %Rotation Method - Arbitrary Axis
  | smiData.RigidTransform(117).translation = [-286.40044094211095 0 0];  % mm
  | smiData.RigidTransform(117).angle = 0;  % rad
  | smiData.RigidTransform(117).axis = [0 0 0];
  | smiData.RigidTransform(117).ID = 'AssemblyGround[tige_verin-4:ecrou-1]';
  | 
  | %Translation Method - Cartesian
  | %Rotation Method - Arbitrary Axis
  | smiData.RigidTransform(118).translation = [-109.40044094211082 0 0];  % mm
  | smiData.RigidTransform(118).angle = 0;  % rad
  | smiData.RigidTransform(118).axis = [0 0 0];
  | smiData.RigidTransform(118).ID = 'AssemblyGround[tige_verin-4:sphere-1]';
  | 
  | 
  | %============= Solid =============%
  | %Center of Mass (CoM) %Moments of Inertia (MoI) %Product of Inertia (PoI)
  | 
  | %Initialize the Solid structure array by filling in null values.
  | smiData.Solid(13).mass = 0.0;
  | smiData.Solid(13).CoM = [0.0 0.0 0.0];
  | smiData.Solid(13).MoI = [0.0 0.0 0.0];
  | smiData.Solid(13).PoI = [0.0 0.0 0.0];
  | smiData.Solid(13).color = [0.0 0.0 0.0];
  | smiData.Solid(13).opacity = 0.0;
  | smiData.Solid(13).ID = '';
  | 
  | %Inertia Type - Custom
  | %Visual Properties - Simple
  | smiData.Solid(1).mass = 0.0084823001646924905;  % kg
  | smiData.Solid(1).CoM = [50.000000000000107 0 0];  % mm
  | smiData.Solid(1).MoI = [1.5480197800563849 7.8425933606052878 7.8425933606052842];  % kg*mm^2
  | smiData.Solid(1).PoI = [0 0 0];  % kg*mm^2
  | smiData.Solid(1).color = [0.5490196078431373 0.88627450980392153 0.37254901960784315];
  | smiData.Solid(1).opacity = 1;
  | smiData.Solid(1).ID = 'tube_inf*:*Defaut';
  | 
  | %Inertia Type - Custom
  | %Visual Properties - Simple
  | smiData.Solid(2).mass = 0.0042139389114065149;  % kg
  | smiData.Solid(2).CoM = [-3.8531148983184531 0 0];  % mm
  | smiData.Solid(2).MoI = [0.3775879875283964 0.38774280929836291 0.38774280929836286];  % kg*mm^2
  | smiData.Solid(2).PoI = [0 0 0];  % kg*mm^2
  | smiData.Solid(2).color = [0.792156862745098 0.81960784313725488 0.93333333333333335];
  | smiData.Solid(2).opacity = 1;
  | smiData.Solid(2).ID = 'embout_inf*:*Defaut';
  | 
  | %Inertia Type - Custom
  | %Visual Properties - Simple
  | smiData.Solid(3).mass = 0.00087691230678662148;  % kg
  | smiData.Solid(3).CoM = [0 0 0];  % mm
  | smiData.Solid(3).MoI = [0.04468468106526724 0.027901923611685846 0.027904881615869789];  % kg*mm^2
  | smiData.Solid(3).PoI = [0 0 1.0399407525185852e-07];  % kg*mm^2
  | smiData.Solid(3).color = [0.792156862745098 0.81960784313725488 0.93333333333333335];
  | smiData.Solid(3).opacity = 1;
  | smiData.Solid(3).ID = 'sphere*:*Defaut';
  | 
  | %Inertia Type - Custom
  | %Visual Properties - Simple
  | smiData.Solid(4).mass = 0.024340536132452913;  % kg
  | smiData.Solid(4).CoM = [-1.7599116330488864 -1.0473499537933795 -2.4933113948030137];  % mm
  | smiData.Solid(4).MoI = [4.7211620239784624 6.4541790251080755 5.1237546606243489];  % kg*mm^2
  | smiData.Solid(4).PoI = [0.10458322744740225 0.11818951483233464 0.044872585268648901];  % kg*mm^2
  | smiData.Solid(4).color = [0.50196078431372548 0.50196078431372548 0.50196078431372548];
  | smiData.Solid(4).opacity = 1;
  | smiData.Solid(4).ID = 'boitier*:*Defaut';
  | 
  | %Inertia Type - Custom
  | %Visual Properties - Simple
  | smiData.Solid(5).mass = 0.016964600329385116;  % kg
  | smiData.Solid(5).CoM = [100.00000000000023 0 0];  % mm
  | smiData.Solid(5).MoI = [3.0960395601127852 58.096687544673458 58.096687544673451];  % kg*mm^2
  | smiData.Solid(5).PoI = [0 0 0];  % kg*mm^2
  | smiData.Solid(5).color = [0.94117647058823528 0.73725490196078436 0.73333333333333328];
  | smiData.Solid(5).opacity = 1;
  | smiData.Solid(5).ID = 'tube_sup*:*Defaut';
  | 
  | %Inertia Type - Custom
  | %Visual Properties - Simple
  | smiData.Solid(6).mass = 0.0090852386604100138;  % kg
  | smiData.Solid(6).CoM = [1.4460647772705237e-05 1.683472159054878e-05 4.9610848302901358];  % mm
  | smiData.Solid(6).MoI = [0.89454060965906912 0.64879030341830701 1.3929994556750713];  % kg*mm^2
  | smiData.Solid(6).PoI = [-5.7536536597541388e-07 -4.8728161404543176e-07 -2.5304487097315138e-08];  % kg*mm^2
  | smiData.Solid(6).color = [0.85882352941176465 0.94901960784313721 0.50196078431372548];
  | smiData.Solid(6).opacity = 1;
  | smiData.Solid(6).ID = 'couvercle*:*Defaut';
  | 
  | %Inertia Type - Custom
  | %Visual Properties - Simple
  | smiData.Solid(7).mass = 0.013822175829353203;  % kg
  | smiData.Solid(7).CoM = [16.32375350866031 0 0];  % mm
  | smiData.Solid(7).MoI = [1.762495070347909 2.4422173514078338 2.4422173514078338];  % kg*mm^2
  | smiData.Solid(7).PoI = [0 0 0];  % kg*mm^2
  | smiData.Solid(7).color = [0.75294117647058822 0.75294117647058822 0.75294117647058822];
  | smiData.Solid(7).opacity = 1;
  | smiData.Solid(7).ID = 'palier*:*Defaut';
  | 
  | %Inertia Type - Custom
  | %Visual Properties - Simple
  | smiData.Solid(8).mass = 0.0025570957599495613;  % kg
  | smiData.Solid(8).CoM = [-5.570192287697922 0 0];  % mm
  | smiData.Solid(8).MoI = [0.0648557791602139 0.15208630974357293 0.15208630974357296];  % kg*mm^2
  | smiData.Solid(8).PoI = [0 0 0];  % kg*mm^2
  | smiData.Solid(8).color = [0.792156862745098 0.81960784313725488 0.93333333333333335];
  | smiData.Solid(8).opacity = 1;
  | smiData.Solid(8).ID = 'embout_sup*:*Defaut';
  | 
  | %Inertia Type - Custom
  | %Visual Properties - Simple
  | smiData.Solid(9).mass = 0.0075398223686154037;  % kg
  | smiData.Solid(9).CoM = [80.000000000000142 0 0];  % mm
  | smiData.Solid(9).MoI = [0.42599996382677108 16.29795436829292 16.29795436829292];  % kg*mm^2
  | smiData.Solid(9).PoI = [0 0 0];  % kg*mm^2
  | smiData.Solid(9).color = [0.792156862745098 0.81960784313725488 0.93333333333333335];
  | smiData.Solid(9).opacity = 1;
  | smiData.Solid(9).ID = 'tige*:*Defaut';
  | 
  | %Inertia Type - Custom
  | %Visual Properties - Simple
  | smiData.Solid(10).mass = 0.004990980951279274;  % kg
  | smiData.Solid(10).CoM = [9.2776978167479065 0.15739895614979629 0];  % mm
  | smiData.Solid(10).MoI = [0.32642178266268096 0.45241671460364152 0.44352864960775157];  % kg*mm^2
  | smiData.Solid(10).PoI = [0 0 0.0053243912629971774];  % kg*mm^2
  | smiData.Solid(10).color = [0.792156862745098 0.81960784313725488 0.93333333333333335];
  | smiData.Solid(10).opacity = 1;
  | smiData.Solid(10).ID = 'ecrou*:*Defaut';
  | 
  | %Inertia Type - Custom
  | %Visual Properties - Simple
  | smiData.Solid(11).mass = 0.0011546366515399924;  % kg
  | smiData.Solid(11).CoM = [0 0 0];  % mm
  | smiData.Solid(11).MoI = [0.10887982247913945 0.059394994553987196 0.059393430668056489];  % kg*mm^2
  | smiData.Solid(11).PoI = [0 0 6.5067408736908672e-09];  % kg*mm^2
  | smiData.Solid(11).color = [0.50196078431372548 0.50196078431372548 1];
  | smiData.Solid(11).opacity = 1;
  | smiData.Solid(11).ID = 'ext_sph*:*Defaut';
  | 
  | %Inertia Type - Custom
  | %Visual Properties - Simple
  | smiData.Solid(12).mass = 0.82140188425764005;  % kg
  | smiData.Solid(12).CoM = [0.00040820266740882615 0.00012122217995162101 1.4602936691808037];  % mm
  | smiData.Solid(12).MoI = [9201.3802380890629 9201.3952989249501 18318.746656983178];  % kg*mm^2
  | smiData.Solid(12).PoI = [-0.00035655541524740205 -0.002943571215792955 -0.015207335347411938];  % kg*mm^2
  | smiData.Solid(12).color = [1 1 0.50196078431372548];
  | smiData.Solid(12).opacity = 1;
  | smiData.Solid(12).ID = 'table3*:*Defaut';
  | 
  | %Inertia Type - Custom
  | %Visual Properties - Simple
  | smiData.Solid(13).mass = 2.2184556724050863;  % kg
  | smiData.Solid(13).CoM = [-0.00038211438954314158 -0.00015795748103623582 16.057226626548466];  % mm
  | smiData.Solid(13).MoI = [46973.417572192877 46973.678310125499 92094.47840429112];  % kg*mm^2
  | smiData.Solid(13).PoI = [-0.015456799387294582 -0.032292544719138144 -0.09445249311157991];  % kg*mm^2
  | smiData.Solid(13).color = [0.50196078431372548 0.50196078431372548 1];
  | smiData.Solid(13).opacity = 1;
  | smiData.Solid(13).ID = 'embase*:*Defaut';
  | 
  | 
  | %============= Joint =============%
  | %X Revolute Primitive (Rx) %Y Revolute Primitive (Ry) %Z Revolute Primitive (Rz)
  | %X Prismatic Primitive (Px) %Y Prismatic Primitive (Py) %Z Prismatic Primitive (Pz) %Spherical Primitive (S)
  | %Constant Velocity Primitive (CV) %Lead Screw Primitive (LS)
  | %Position Target (Pos)
  | 
  | %Initialize the CylindricalJoint structure array by filling in null values.
  | smiData.CylindricalJoint(6).Rz.Pos = 0.0;
  | smiData.CylindricalJoint(6).Pz.Pos = 0.0;
  | smiData.CylindricalJoint(6).ID = '';
  | 
  | smiData.CylindricalJoint(1).Rz.Pos = -104.20003358622741;  % deg
  | smiData.CylindricalJoint(1).Pz.Pos = 0;  % mm
  | smiData.CylindricalJoint(1).ID = '[corps_verin-1:-:tige_verin-1]';
  | 
  | smiData.CylindricalJoint(2).Rz.Pos = -37.792584245206498;  % deg
  | smiData.CylindricalJoint(2).Pz.Pos = 0;  % mm
  | smiData.CylindricalJoint(2).ID = '[corps_verin-2:-:tige_verin-2]';
  | 
  | smiData.CylindricalJoint(3).Rz.Pos = -42.310579847602945;  % deg
  | smiData.CylindricalJoint(3).Pz.Pos = 0;  % mm
  | smiData.CylindricalJoint(3).ID = '[corps_verin-3:-:tige_verin-4]';
  | 
  | smiData.CylindricalJoint(4).Rz.Pos = -140.18477551834167;  % deg
  | smiData.CylindricalJoint(4).Pz.Pos = 0;  % mm
  | smiData.CylindricalJoint(4).ID = '[corps_verin-4:-:tige_verin-5]';
  | 
  | smiData.CylindricalJoint(5).Rz.Pos = -53.160272688945668;  % deg
  | smiData.CylindricalJoint(5).Pz.Pos = 0;  % mm
  | smiData.CylindricalJoint(5).ID = '[corps_verin-5:-:tige_verin-6]';
  | 
  | smiData.CylindricalJoint(6).Rz.Pos = -4.4711393322405737;  % deg
  | smiData.CylindricalJoint(6).Pz.Pos = 0;  % mm
  | smiData.CylindricalJoint(6).ID = '[corps_verin-6:-:tige_verin-7]';
  | 
  | 
  | %Initialize the SphericalJoint structure array by filling in null values.
  | smiData.SphericalJoint(12).S.Pos.Angle = 0.0;
  | smiData.SphericalJoint(12).S.Pos.Axis = [0.0 0.0 0.0];
  | smiData.SphericalJoint(12).ID = '';
  | 
  | smiData.SphericalJoint(1).S.Pos.Angle = 81.540514948179705;  % deg
  | smiData.SphericalJoint(1).S.Pos.Axis = [-0.050833017106464505 -0.85475299427067353 0.51653975951244224];
  | smiData.SphericalJoint(1).ID = '[tige_verin-1:-:table_pltf-1]';
  | 
  | %This joint has been chosen as a cut joint. Simscape Multibody treats cut joints as algebraic constraints to solve closed kinematic loops. The imported model does not use the state target data for this joint.
  | smiData.SphericalJoint(2).S.Pos.Angle = 122.12501049103869;  % deg
  | smiData.SphericalJoint(2).S.Pos.Axis = [-0.8108109832772139 -0.37416290793533363 0.45009739804003823];
  | smiData.SphericalJoint(2).ID = '[tige_verin-2:-:table_pltf-1]';
  | 
  | %This joint has been chosen as a cut joint. Simscape Multibody treats cut joints as algebraic constraints to solve closed kinematic loops. The imported model does not use the state target data for this joint.
  | smiData.SphericalJoint(3).S.Pos.Angle = 120.19250825600254;  % deg
  | smiData.SphericalJoint(3).S.Pos.Axis = [0.094584503624073835 -0.95986821412891099 -0.26402042189793368];
  | smiData.SphericalJoint(3).ID = '[tige_verin-4:-:table_pltf-1]';
  | 
  | %This joint has been chosen as a cut joint. Simscape Multibody treats cut joints as algebraic constraints to solve closed kinematic loops. The imported model does not use the state target data for this joint.
  | smiData.SphericalJoint(4).S.Pos.Angle = 112.46403356373973;  % deg
  | smiData.SphericalJoint(4).S.Pos.Axis = [0.39724751293372007 -0.91701725047696303 -0.035689995736126551];
  | smiData.SphericalJoint(4).ID = '[tige_verin-5:-:table_pltf-1]';
  | 
  | %This joint has been chosen as a cut joint. Simscape Multibody treats cut joints as algebraic constraints to solve closed kinematic loops. The imported model does not use the state target data for this joint.
  | smiData.SphericalJoint(5).S.Pos.Angle = 132.67550049039835;  % deg
  | smiData.SphericalJoint(5).S.Pos.Axis = [0.77328833426052934 -0.078395523841644235 -0.62918939433064991];
  | smiData.SphericalJoint(5).ID = '[tige_verin-6:-:table_pltf-1]';
  | 
  | %This joint has been chosen as a cut joint. Simscape Multibody treats cut joints as algebraic constraints to solve closed kinematic loops. The imported model does not use the state target data for this joint.
  | smiData.SphericalJoint(6).S.Pos.Angle = 110.12939777928017;  % deg
  | smiData.SphericalJoint(6).S.Pos.Axis = [0.12182095314015672 -0.83924823324724662 -0.52992646505661412];
  | smiData.SphericalJoint(6).ID = '[tige_verin-7:-:table_pltf-1]';
  | 
  | smiData.SphericalJoint(7).S.Pos.Angle = 114.02300404344669;  % deg
  | smiData.SphericalJoint(7).S.Pos.Axis = [-0.23835760860008021 0.96972202683315023 -0.053149234209514923];
  | smiData.SphericalJoint(7).ID = '[embase_pltf-1:-:corps_verin-1]';
  | 
  | smiData.SphericalJoint(8).S.Pos.Angle = 124.36289440834484;  % deg
  | smiData.SphericalJoint(8).S.Pos.Axis = [0.75127480367294575 0.13666963532919338 -0.64568380817948512];
  | smiData.SphericalJoint(8).ID = '[embase_pltf-1:-:corps_verin-2]';
  | 
  | smiData.SphericalJoint(9).S.Pos.Angle = 101.04923269288062;  % deg
  | smiData.SphericalJoint(9).S.Pos.Axis = [0.154512695452697 0.94279726439292089 0.29539658968438831];
  | smiData.SphericalJoint(9).ID = '[embase_pltf-1:-:corps_verin-3]';
  | 
  | smiData.SphericalJoint(10).S.Pos.Angle = 150.30973644815009;  % deg
  | smiData.SphericalJoint(10).S.Pos.Axis = [-0.45431151675831594 0.53547234394518495 0.71194832299163957];
  | smiData.SphericalJoint(10).ID = '[embase_pltf-1:-:corps_verin-4]';
  | 
  | smiData.SphericalJoint(11).S.Pos.Angle = 144.25978030466871;  % deg
  | smiData.SphericalJoint(11).S.Pos.Axis = [-0.84495140385431233 0.24792317573491993 0.47391056546371574];
  | smiData.SphericalJoint(11).ID = '[embase_pltf-1:-:corps_verin-5]';
  | 
  | smiData.SphericalJoint(12).S.Pos.Angle = 87.070863293138117;  % deg
  | smiData.SphericalJoint(12).S.Pos.Axis = [0.32601675830399962 0.93004557939395283 0.16949422867672598];
  | smiData.SphericalJoint(12).ID = '[embase_pltf-1:-:corps_verin-6]';
undefined symbols (not defined in the file or in its folder): smiData, X, Y, Z
libraries: sm_lib x329, nesl_utility x19
(part 1 of 7)
settings Model: Creator=Renaud  LastModifiedBy=Renaud

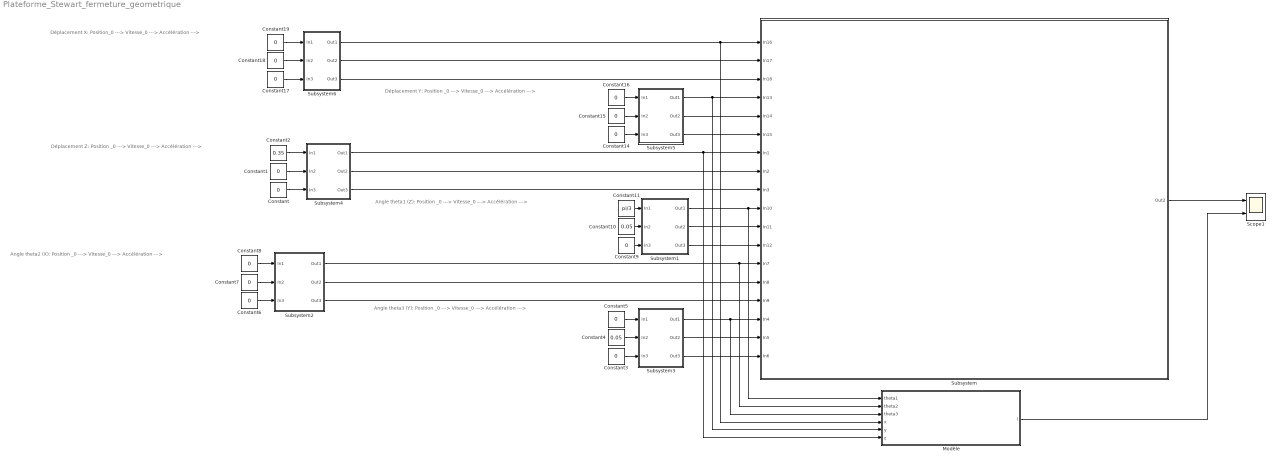
== system Plateforme_Stewart_fermeture_geometrique ==
  note: Angle theta3 (Y):	Position	_0		--->
      | 											Vitesse_0		--->
      | 											Accélération	--->
  note: Angle theta2 (X):	Position	_0		--->
      | 											Vitesse_0		--->
      | 											Accélération	--->
  note: Angle theta1 (Z):	Position	_0		--->
      | 											Vitesse_0		--->
      | 											Accélération	--->
  note: Déplacement Z:	Position	_0		--->
      | 										Vitesse_0		--->
      | 										Accélération	--->
  note: Déplacement Y:	Position	_0		--->
      | 										Vitesse_0		--->
      | 										Accélération	--->
  note: Déplacement X:	Position_0		--->
      | 										Vitesse_0		--->
      | 										Accélération	--->
  Constant{,1,3,5..9,14..19} (14 alike) : Constant  Value=0
  Constant10 : Constant  Value=0.05
  Constant11 : Constant  Value=pi/3
  Constant2 : Constant  Value=0.35
  Constant4 : Constant  Value=0.05
  Modèle : MATLAB Function  TreatAsAtomicUnit=on
  Scope1 : Scope  NumInputPorts=2
  Subsystem : Subsystem
      mask Display: image('$imagefile'); % Use "Edit Image" on toolstrip to change.
  Subsystem1 : Subsystem
  Subsystem2 : Subsystem
  Subsystem3 : Subsystem
  Subsystem4 : Subsystem
  Subsystem5 : Subsystem
  Subsystem6 : Subsystem
  wires:
  Constant3/1 -> Subsystem3/3(In3)
  Constant9/1 -> Subsystem1/3(In3)
  Constant6/1 -> Subsystem2/3(In3)
  Subsystem6/1(Out1) -> Modèle/4(x), Subsystem/1(In16)
  Subsystem5/1(Out1) -> Modèle/5(y), Subsystem/4(In13)
  Subsystem1/1(Out1) -> Modèle/1(theta1), Subsystem/10(In10)
  Constant11/1 -> Subsystem1/1(In1)
  Constant10/1 -> Subsystem1/2(In2)
  Subsystem1/2(Out2) -> Subsystem/11(In11)
  Subsystem2/1(Out1) -> Modèle/2(theta2), Subsystem/13(In7)
  Constant8/1 -> Subsystem2/1(In1)
  Constant7/1 -> Subsystem2/2(In2)
  Subsystem2/2(Out2) -> Subsystem/14(In8)
  Constant5/1 -> Subsystem3/1(In1)
  Constant4/1 -> Subsystem3/2(In2)
  Subsystem3/2(Out2) -> Subsystem/17(In5)
  Subsystem4/1(Out1) -> Modèle/6(z), Subsystem/7(In1)
  Constant2/1 -> Subsystem4/1(In1)
  Constant1/1 -> Subsystem4/2(In2)
  Constant/1 -> Subsystem4/3(In3)
  Subsystem4/2(Out2) -> Subsystem/8(In2)
  Subsystem4/3(Out3) -> Subsystem/9(In3)
  Constant15/1 -> Subsystem5/2(In2)
  Constant14/1 -> Subsystem5/3(In3)
  Constant16/1 -> Subsystem5/1(In1)
  Constant18/1 -> Subsystem6/2(In2)
  Constant17/1 -> Subsystem6/3(In3)
  Constant19/1 -> Subsystem6/1(In1)
  Subsystem6/2(Out2) -> Subsystem/2(In17)
  Subsystem6/3(Out3) -> Subsystem/3(In18)
  Subsystem5/2(Out2) -> Subsystem/5(In14)
  Subsystem5/3(Out3) -> Subsystem/6(In15)
  Subsystem3/3(Out3) -> Subsystem/18(In6)
  Subsystem2/3(Out3) -> Subsystem/15(In9)
  Subsystem1/3(Out3) -> Subsystem/12(In12)
  Subsystem3/1(Out1) -> Modèle/3(theta3), Subsystem/16(In4)
  Modèle/1(l) -> Scope1/2
  Subsystem/1(Out2) -> Scope1/1
